simulink model "ScopeMultiRate"  (R2024b)
settings: Solver=VariableStepAuto  StartTime=0.0  StopTime=0.4  FixedStep=.01  RelTol=1e-3
settings Model: Creator=The MathWorks, Inc.  LastModifiedBy=The MathWorks, Inc.
settings DebuggingCC: UnconnectedInputMsg=warning  UnconnectedOutputMsg=warning  UnconnectedLineMsg=warning
settings ModelReferenceCC: EnableRefExpFcnMdlSchedulingChecks=on
settings RTWCC: GPUComputeCapability=3.5  DLArmComputeVersion=19.05

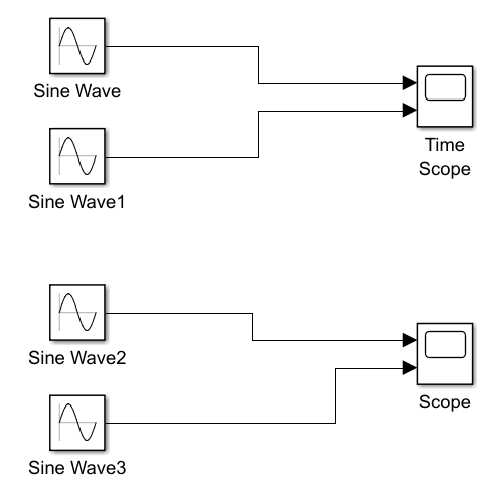
[thumbnail: Simulink's stored preview of the top-level diagram]
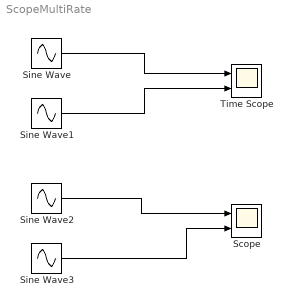
== system ScopeMultiRate ==
  Scope : Scope  NumInputPorts=2
  Sine Wave{,1..3} (4 alike) : Sin  Frequency=100
  Time Scope : Scope  NumInputPorts=2
  wires:
  Sine Wave2/1 -> Scope/1
  Sine Wave3/1 -> Scope/2
  Sine Wave1/1 -> Time Scope/2
  Sine Wave/1 -> Time Scope/1
